simulink model "backstepping"  (R2017a)
settings: Solver=VariableStepAuto  StartTime=0.0  StopTime=10.0  RelTol=1e-3
model workspace: external: MAT-File R:\ggdrive\code\Matlab\QuadSim\Simulink\full_model\parameters\param.mat (data not in the file)
settings Model: Creator=calvinv  LastModifiedBy=calvin

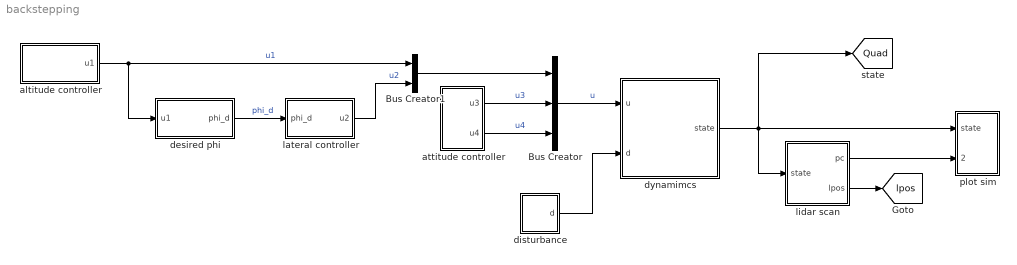
== system backstepping ==
  Bus Creator : BusCreator  Inputs=3
  Bus Creator1 : BusCreator  Inputs=2
  altitude controller : Subsystem  mask{k1=5, k2=5, zd=1.5}
      mask prompts: zd "desired z"
  attitude controller : Subsystem  mask{P_the=1, D_the=1.5, P_psi=1, D_psi=1.5}
      mask prompts: P_the "Theta P gain"; D_the "Theta D gain"; P_psi "Psi P gain"; D_psi "Pis D gain"
      mask DialogControl DescGroupVar Prompt: Attitude PD controller
  desired phi : Subsystem  mask{k3=1, k4=1, yd=-1}
      mask prompts: yd "desired y"
  disturbance : Subsystem  mask{freq=20, amp1=5, amp_f=2, amp_tau=0, amp_tau_freq=0, tau_freq=5}
      mask prompts: freq "force oscillation freq"; amp1 "Force amplitude"; amp_f "force oscillation amplitude"; amp_tau "Torque disturbance amplitude"; amp_tau_freq "Torque oscillation freq amp"; tau_freq "Torque oscillation freq"
      mask DialogControl DescGroupVar Prompt: Disturbance generator
  dynamimcs : Subsystem
  lateral controller : Subsystem  mask{P=40, D=9}
      mask DialogControl DescGroupVar Prompt: Attitude PD controller
  lidar scan : Subsystem
  plot sim : Subsystem
  tag scope: Quad=global, lpos=global
  wires:
  attitude controller/1(u3) -> Bus Creator/2  "u3"
  disturbance/1(d) -> dynamimcs/2(d)
  lidar scan/1(pc) -> plot sim/2(lidar pc)
  attitude controller/2("u4 ") -> Bus Creator/3  "u4"
  Bus Creator/1 -> dynamimcs/1(u)  "u"
  lidar scan/2(lpos) -> [lpos]
  dynamimcs/1(state) -> lidar scan/1(state), plot sim/1(state), [Quad]
  altitude controller/1(u1) -> desired phi/1(u1), Bus Creator1/1  "u1"
  Bus Creator1/1 -> Bus Creator/1
  lateral controller/1(u2) -> Bus Creator1/2  "u2"
  desired phi/1(phi_d) -> lateral controller/1(phi_d)  "phi_d"

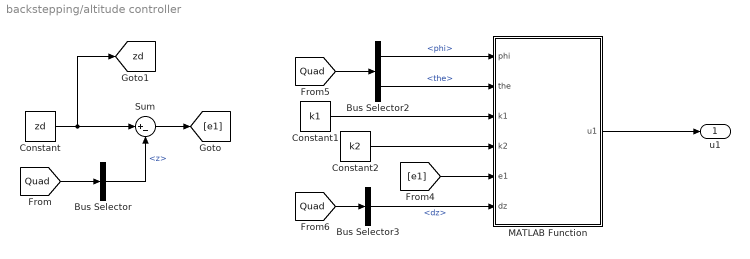
== system backstepping/altitude controller ==
  Bus Selector : BusSelector  OutputSignals=z
  Bus Selector2 : BusSelector  OutputSignals=phi,the
  Bus Selector3 : BusSelector  OutputSignals=dz
  Constant : Constant  Value=zd
  Constant1 : Constant  Value=k1
  Constant2 : Constant  Value=k2
  MATLAB Function : MATLAB Function  TreatAsAtomicUnit=on
  Sum : Sum  Inputs=|+-
  u1 : Outport
  tag scope: zd=global
  wires:
  [Quad] -> Bus Selector/1
  Constant/1 -> [zd], Sum/1
  Bus Selector/1 -> Sum/2  "<z>"
  Sum/1 -> [e1]
  [e1] -> MATLAB Function/5(e1)
  [Quad] -> Bus Selector2/1
  Bus Selector2/1 -> MATLAB Function/1(phi)  "<phi>"
  Bus Selector2/2 -> MATLAB Function/2(the)  "<the>"
  Constant1/1 -> MATLAB Function/3(k1)
  Constant2/1 -> MATLAB Function/4(k2)
  Bus Selector3/1 -> MATLAB Function/6(dz)  "<dz>"
  [Quad] -> Bus Selector3/1
  MATLAB Function/1(u1) -> u1/1

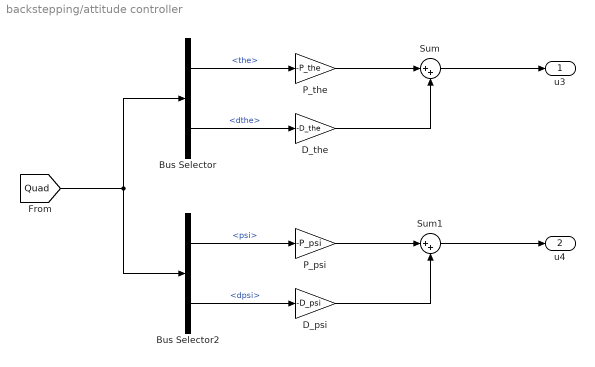
== system backstepping/attitude controller ==
  Bus Selector : BusSelector  OutputSignals=the,dthe
  Bus Selector2 : BusSelector  OutputSignals=psi,dpsi
  D_psi : Gain  Gain=-D_psi
  D_the : Gain  Gain=-D_the
  P_psi : Gain  Gain=-P_psi
  P_the : Gain  Gain=-P_the
  Sum : Sum  Inputs=|++
  Sum1 : Sum  Inputs=|++
  u3 : Outport
  "u4 " : Outport  Port=2
  wires:
  [Quad] -> Bus Selector2/1, Bus Selector/1
  D_the/1 -> Sum/2
  P_the/1 -> Sum/1
  Bus Selector/2 -> D_the/1  "<dthe>"
  Bus Selector/1 -> P_the/1  "<the>"
  Sum/1 -> u3/1
  Bus Selector2/1 -> P_psi/1  "<psi>"
  Bus Selector2/2 -> D_psi/1  "<dpsi>"
  P_psi/1 -> Sum1/1
  D_psi/1 -> Sum1/2
  Sum1/1 -> "u4 "/1

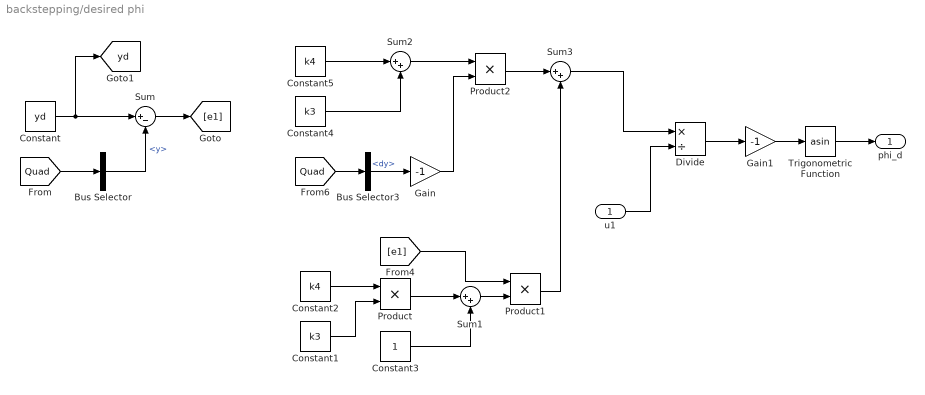
== system backstepping/desired phi ==
  u1 : Inport
  Bus Selector : BusSelector  OutputSignals=y
  Bus Selector3 : BusSelector  OutputSignals=dy
  Constant : Constant  Value=yd
  Constant1 : Constant  Value=k3
  Constant2 : Constant  Value=k4
  Constant3 : Constant
  Constant4 : Constant  Value=k3
  Constant5 : Constant  Value=k4
  Divide : Product  Inputs=*/
  Gain : Gain  Gain=-1
  Gain1 : Gain  Gain=-1
  Product : Product
  Product1 : Product
  Product2 : Product
  Sum : Sum  Inputs=|+-
  Sum1 : Sum  Inputs=|++
  Sum2 : Sum  Inputs=|++
  Sum3 : Sum  Inputs=|++
  Trigonometric Function : Trigonometry  Operator=asin
  phi_d : Outport
  tag scope: yd=global
  wires:
  [Quad] -> Bus Selector3/1
  Sum/1 -> [e1]
  Bus Selector/1 -> Sum/2  "<y>"
  Constant/1 -> [yd], Sum/1
  [Quad] -> Bus Selector/1
  u1/1 -> Divide/2
  Constant2/1 -> Product/1
  Constant1/1 -> Product/2
  Product/1 -> Sum1/1
  Constant3/1 -> Sum1/2
  Sum1/1 -> Product1/2
  [e1] -> Product1/1
  Constant5/1 -> Sum2/1
  Constant4/1 -> Sum2/2
  Sum2/1 -> Product2/1
  Bus Selector3/1 -> Gain/1  "<dy>"
  Gain/1 -> Product2/2
  Product2/1 -> Sum3/1
  Product1/1 -> Sum3/2
  Sum3/1 -> Divide/1
  Divide/1 -> Gain1/1
  Trigonometric Function/1 -> phi_d/1
  Gain1/1 -> Trigonometric Function/1

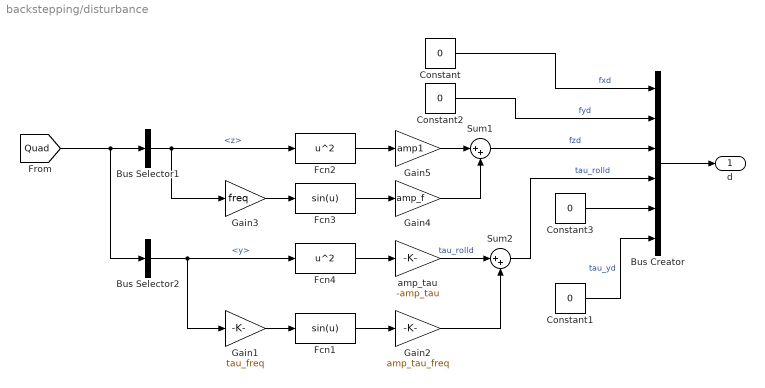
== system backstepping/disturbance ==
  Bus Creator : BusCreator  Inputs=6
  Bus Selector1 : BusSelector  OutputSignals=z
  Bus Selector2 : BusSelector  OutputSignals=y
  Constant{,1..3} (4 alike) : Constant  Value=0
  Fcn1 : Fcn  Expr=sin(u)
  Fcn2 : Fcn  Expr=u^2
  Fcn3 : Fcn  Expr=sin(u)
  Fcn4 : Fcn  Expr=u^2
  Gain1 : Gain  Gain=tau_freq
  Gain2 : Gain  Gain=amp_tau_freq
  Gain3 : Gain  Gain=freq
  Gain4 : Gain  Gain=amp_f
  Gain5 : Gain  Gain=amp1
  Sum1 : Sum  Inputs=|++
  Sum2 : Sum  Inputs=|++
  amp_tau : Gain  Gain=-amp_tau
  d : Outport
  wires:
  [Quad] -> Bus Selector2/1, Bus Selector1/1
  Gain4/1 -> Sum1/2
  Gain5/1 -> Sum1/1
  Bus Selector1/1 -> Fcn2/1, Gain3/1  "<z>"
  Fcn2/1 -> Gain5/1
  Fcn3/1 -> Gain4/1
  Gain3/1 -> Fcn3/1
  Constant2/1 -> Bus Creator/2  "fyd"
  Sum1/1 -> Bus Creator/3  "fzd"
  Constant/1 -> Bus Creator/1  "fxd"
  Bus Creator/1 -> d/1
  Constant1/1 -> Bus Creator/6  "tau_yd"
  Fcn4/1 -> amp_tau/1
  Bus Selector2/1 -> Gain1/1, Fcn4/1  "<y>"
  Gain1/1 -> Fcn1/1
  Fcn1/1 -> Gain2/1
  amp_tau/1 -> Sum2/1  "tau_rolld"
  Gain2/1 -> Sum2/2
  Sum2/1 -> Bus Creator/4  "tau_rolld"
  Constant3/1 -> Bus Creator/5

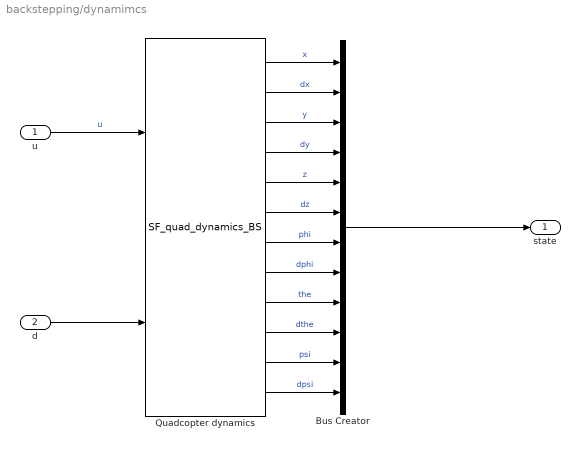
== system backstepping/dynamimcs ==
  u : Inport
  d : Inport  Port=2
  Bus Creator : BusCreator  Inputs=12
  Quadcopter dynamics : M-S-Function  FunctionName=SF_quad_dynamics_BS  Parameters=quad
  state : Outport
  wires:
  Bus Creator/1 -> state/1
  u/1 -> Quadcopter dynamics/1  "u"
  d/1 -> Quadcopter dynamics/2
  Quadcopter dynamics/1 -> Bus Creator/1  "x"
  Quadcopter dynamics/2 -> Bus Creator/2  "dx"
  Quadcopter dynamics/3 -> Bus Creator/3  "y"
  Quadcopter dynamics/4 -> Bus Creator/4  "dy"
  Quadcopter dynamics/5 -> Bus Creator/5  "z"
  Quadcopter dynamics/6 -> Bus Creator/6  "dz"
  Quadcopter dynamics/7 -> Bus Creator/7  "phi"
  Quadcopter dynamics/8 -> Bus Creator/8  "dphi"
  Quadcopter dynamics/9 -> Bus Creator/9  "the"
  Quadcopter dynamics/10 -> Bus Creator/10  "dthe"
  Quadcopter dynamics/11 -> Bus Creator/11  "psi"
  Quadcopter dynamics/12 -> Bus Creator/12  "dpsi"

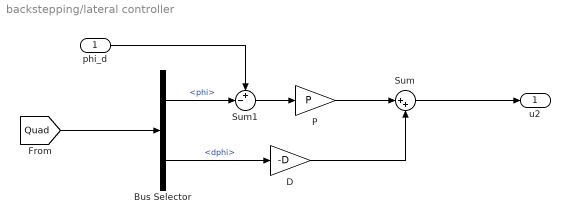
== system backstepping/lateral controller ==
  phi_d : Inport
  Bus Selector : BusSelector  OutputSignals=phi,dphi
  D : Gain  Gain=-D
  P : Gain  Gain=P
  Sum : Sum  Inputs=|++
  Sum1 : Sum  Inputs=+-|
  u2 : Outport
  wires:
  Sum/1 -> u2/1
  Bus Selector/2 -> D/1  "<dphi>"
  P/1 -> Sum/1
  D/1 -> Sum/2
  [Quad] -> Bus Selector/1
  Bus Selector/1 -> Sum1/2  "<phi>"
  Sum1/1 -> P/1
  phi_d/1 -> Sum1/1

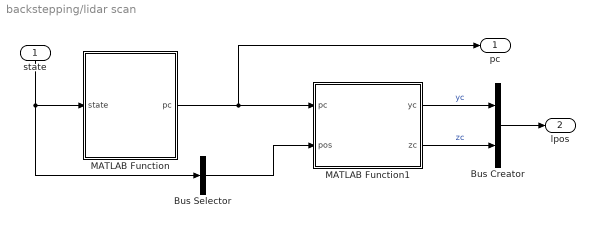
== system backstepping/lidar scan ==
  state : Inport
  Bus Creator : BusCreator  Inputs=2
  Bus Selector : BusSelector  OutputSignals=y,z  OutputAsBus=on
  MATLAB Function : MATLAB Function  TreatAsAtomicUnit=on
  MATLAB Function1 : MATLAB Function  TreatAsAtomicUnit=on
  pc : Outport
  lpos : Outport  Port=2
  wires:
  state/1 -> MATLAB Function/1(state), Bus Selector/1
  MATLAB Function/1(pc) -> pc/1, MATLAB Function1/1(pc)
  Bus Selector/1 -> MATLAB Function1/2(pos)
  MATLAB Function1/1(yc) -> Bus Creator/1  "yc"
  MATLAB Function1/2(zc) -> Bus Creator/2  "zc"
  Bus Creator/1 -> lpos/1

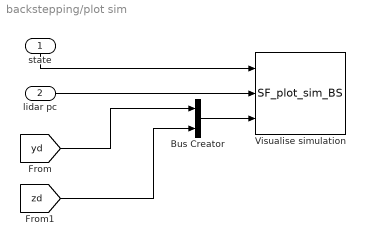
== system backstepping/plot sim ==
  state : Inport
  lidar pc : Inport  Port=2
  Bus Creator : BusCreator  Inputs=2
  "Visualise simulation " : M-S-Function  FunctionName=SF_plot_sim_BS  Parameters=quad
  wires:
  state/1 -> "Visualise simulation "/1
  lidar pc/1 -> "Visualise simulation "/2
  Bus Creator/1 -> "Visualise simulation "/3
  [yd] -> Bus Creator/1
  [zd] -> Bus Creator/2

== matlab function backstepping/altitude controller/MATLAB Function ==
  data: phi input; u1 output; the input; k1 input; k2 input; e1 input; dz input
function u1 = ctrl_law(phi, the, k1, k2, e1, dz)

u1 = (9.81 + 0 - (k1+k2)*dz + (1+k1*k2)*e1)/(cos(phi)*cos(the)) ;

== matlab function backstepping/lidar scan/MATLAB Function ==
  data: state input; pc output
%% need another and condition inside wall check


function pc = lidar_scan_gen(state)

%% init
tunnel_r = 1.5;
tunnel_l = 6; % tunnel length;

a = -135:0.25:135; % lidar FOV is 270 deg

a = a .* pi/180;

pc = zeros(length(a)+5, 3);
temp = zeros(length(a), 3);

z_ceiling = 2 * tunnel_r;
z_ground = 0;

wall_left = -tunnel_r;
wall_right = tunnel_r;

pos_x = state(1);
pos_y = state(3);
pos_z = state(5);
phi = state(7);
the = state(9);
psi = state(11);
the = 0;
psi = 0;

%% checking intersection 
np = 1;
c = 1;
oline = zeros(5,3);

for m = 1:length(a)
    
    angle = [phi the psi];
    
    % generate line point
    r = 20*tunnel_r;
    p = [0 r*sin(a(m)) r*cos(a(m))]';

    pos = [pos_x pos_y pos_z]; % position of the quad
    
    p = Rzyx(angle) * p + pos';    % apply rotation
    
    % wall planes - top right bot left
    n = [0 0 1;0 1 0;0 0 1;0 -1 0];
    wall0 = [0 0 z_ceiling;0 wall_right 0;0 0 z_ground;0 wall_left 0];
    
    for b = 1:4
        [p_wall,check] = plane_line_intersect(n(b, :), wall0(b, :) ,pos ,p');

        if check == 1
            if round(p_wall(2)*1e10)/1e10 > wall_right || round(p_wall(2)*1e10)/1e10 < wall_left
                continue;
            elseif round(p_wall(3)*1e10)/1e10 > z_ceiling || round(p_wall(3)*1e10)/1e10 < z_ground   
                continue;
            else
                break;
            end
        end
    end
    
    % oline is for plotting the centre lines
    
    if m == 1 || m == 1081 || m == 1080/2 || m == 180 || m == 1081-180
        oline(c,:) = p_wall;
        c = c + 1;
    end
    
    lidar_noise = [0 50 - randi(100,1) 50-randi(100,1)]./1000;  % +/- 50mm noise
    
    temp(np,:) = p_wall+ lidar_noise;
    np = np + 1;
end

pc = [oline;temp];

end

== matlab function backstepping/lidar scan/MATLAB Function1 ==
  data: pc input; yc output; pos input; zc output
function [yc, zc] = get_centroid(pc, pos)

% init
pc = pc(6:end, :);
A = 0;
cy = 0;
cz = 0;

py = pos(1);
pz = pos(2);



y = pc(:,2) + py;
z = pc(:,3) + pz -1.5;

for n = 1:length(pc)-1

    A = A + (y(n) * z(n+1)) - (y(n+1) * z(n));

    cy = cy + (y(n) + y(n+1)) * (y(n) * z(n+1) - y(n+1) * z(n));
    cz = cz + (z(n) + z(n+1)) * (y(n) * z(n+1) - y(n+1) * z(n));
  
end

A = A/2;


pos_loc_y2 = cy/(6 * A);
pos_loc_z2 = cz/(6 * A);



A = -A/(1000^2);
area = A;

yc = pos_loc_y2;
zc = pos_loc_z2;
